simulink model "dynamiczny_model_dyskretny"  (R2016b)
settings: Solver=ode45  StartTime=0.0  StopTime=100  RelTol=1e-3  EnableMultiTasking=on
values from neighbouring files (symbols this model uses):
  a1 = -0.19    [initial.m]
  a2 = -0.05    [initial.m]
  a3 = -0.95    [initial.m]
  a4 = -0.45    [initial.m]
  T1 = 7    [initial.m]
  T2 = 7    [initial.m]
  Tp = 2    [initial.m]
settings Model: Creator=Agnieszka i Kamilka  LastModifiedBy=kamil
settings DataIOCC: LimitDataPoints=on  SaveFormat=Array  SignalLoggingSaveFormat=ModelDataLogs
settings OptimizationCC: ExpressionDepthLimit=2147483647  LifeSpan=inf
settings DebuggingCC: UnderspecifiedInitializationDetection=Classic  MergeDetectMultiDrivingBlocksExec=none  SolverPrmCheckMsg=warning  FcnCallInpInsideContextMsg=warning  StateNameClashWarn=warning  SFUnexpectedBacktrackingDiag=warning  SFNoUnconditionalDefaultTransitionDiag=warning  SFExecutionAtInitializationDiag=none
settings HardwareCC: ProdBitPerPointer=32  ProdBitPerSizeT=32  ProdBitPerPtrDiffT=32  ProdLargestAtomicFloat=None  ProdIntDivRoundTo=Undefined  ProdEndianess=Unspecified  ProdWordSize=32  ProdHWDeviceType=32-bit Generic
settings ModelReferenceCC: PropagateSignalLabelsOutOfModel=off
settings GRTTargetCC: TargetLangStandard=C89/C90 (ANSI)  GeneratePreprocessorConditionals=Disable all  CombineOutputUpdateFcns=off  GRTInterface=on
settings ConfigComp: CovMetricSettings=dw  CovHtmlReporting=on  CovSaveCumulativeToWorkspaceVar=on  CovSaveSingleToWorkspaceVar=on  CovExternalEMLEnable=off

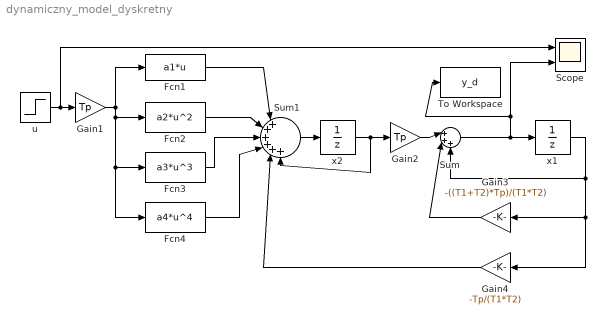
== system dynamiczny_model_dyskretny ==
  Fcn1 : Fcn  Expr=a1*u
  Fcn2 : Fcn  Expr=a2*u^2
  Fcn3 : Fcn  Expr=a3*u^3
  Fcn4 : Fcn  Expr=a4*u^4
  "Gain1 " : Gain  Gain=Tp
  Gain2 : Gain  Gain=Tp
  Gain3 : Gain  Gain=-((T1+T2)*Tp)/(T1*T2)
  Gain4 : Gain  Gain=-Tp/(T1*T2)
  Scope : Scope  NumInputPorts=2
  Sum : Sum  Inputs=|+++
  Sum1 : Sum  Inputs=|++++++
  To Workspace : ToWorkspace  VariableName=y_d  SaveFormat=Structure With Time  SampleTime=-1
  u : Step  SampleTime=0
  x1 : UnitDelay  SampleTime=-1
  x2 : UnitDelay  SampleTime=-1
  wires:
  Sum/1 -> x1/1, Scope/2, To Workspace/1
  Gain2/1 -> Sum/1
  x2/1 -> Gain2/1, Sum1/6
  Gain3/1 -> Sum/2
  u/1 -> Scope/1, "Gain1 "/1
  "Gain1 "/1 -> Fcn1/1, Fcn4/1, Fcn3/1, Fcn2/1
  Fcn1/1 -> Sum1/1
  Fcn2/1 -> Sum1/2
  Fcn3/1 -> Sum1/3
  Fcn4/1 -> Sum1/4
  Sum1/1 -> x2/1
  Gain4/1 -> Sum1/5
  x1/1 -> Sum/3, Gain3/1, Gain4/1
